simulink model "simLink_linefollower"  (R2022b)
settings: Solver=FixedStepAuto  StartTime=0.0  StopTime=10  FixedStep=0.1  RelTol=1e-3
values from neighbouring files (symbols this model uses):
  length_body = pixel_body/pixel_conversion    (= 80)    [startSim.m]
  length_close_sensor = pixel_body/pixel_conversion    (= 80)    [startSim.m]
  map = zeros(map_size_x, map_size_y)    [generate_map.m]    (also in startSim.m = imcomplement(map))
  pixel_sensor = 3    [startSim.m]
  Position_noise = 0    [startSim.m]
  reading_noise = 0    [startSim.m]
  spacing = 2/pixel_conversion    (= 20)    [startSim.m]
  velocity_left = 80    [startSim.m]
  velocity_right = 80    [startSim.m]
undefined symbols (not defined in the file or in its folder): offset_x, offset_y
libraries: simulink x28, slpidlib x1, robotmobilelib x1
(part 1 of 2)
settings Model: Creator=andre  LastModifiedBy=andre

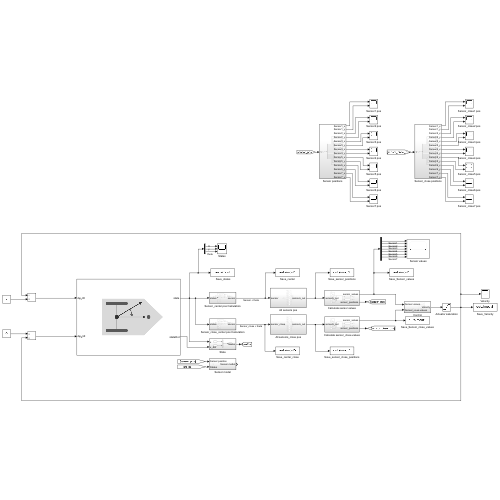
[thumbnail: Simulink's stored preview of the top-level diagram]
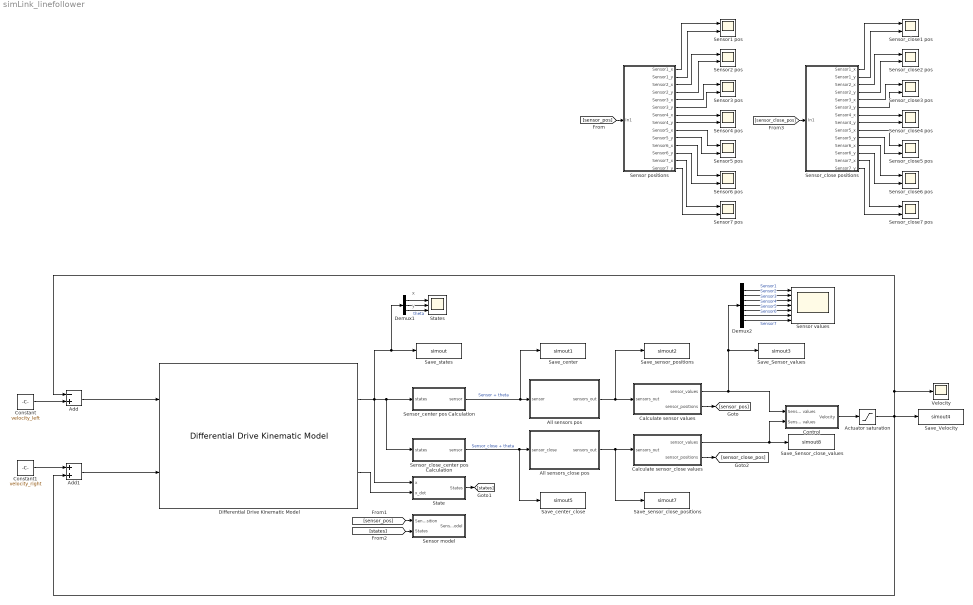
== system simLink_linefollower ==
  note: y
  note: x
  " Save_states" : ToWorkspace  VariableName=simout  SaveFormat=Structure With Time  SampleTime=-1
  Actuator saturation : Saturate  UpperLimit=velocity_left*2  LowerLimit=-velocity_left*2
  Add : Sum  Inputs=-+
  Add1 : Sum
  All sensors pos : Subsystem
  All sensors_close pos : Subsystem
  Calculate sensor values : Subsystem
  Calculate sensor_close values : Subsystem
  Constant : Constant  Value=velocity_left
  Constant1 : Constant  Value=velocity_right
  Control : Subsystem
  Demux1 : Demux  Outputs=3
  Demux2 : Demux  Outputs=7
  Differential Drive Kinematic Model : robotmobilelib/Differential Drive Kinematic Model  VehicleInputs=Wheel Speeds  WheelRadius=length_body*0.1  WheelSpeedRange=[-inf inf]  TrackWidth=length_body*0.7  InitialState=initialState  SimulateUsing=Interpreted execution
  Save_Sensor_close_values : ToWorkspace  VariableName=simout8  SaveFormat=Structure With Time  SampleTime=-1
  Save_Sensor_values : ToWorkspace  VariableName=simout3  SaveFormat=Structure With Time  SampleTime=-1
  Save_Velocity : ToWorkspace  VariableName=simout4  SaveFormat=Structure With Time  SampleTime=-1
  Save_center : ToWorkspace  VariableName=simout1  SaveFormat=Structure With Time  SampleTime=-1
  Save_center_close : ToWorkspace  VariableName=simout5  SaveFormat=Structure With Time  SampleTime=-1
  Save_sensor_close_positions : ToWorkspace  VariableName=simout7  SaveFormat=Structure With Time  SampleTime=-1
  Save_sensor_positions : ToWorkspace  VariableName=simout2  SaveFormat=Structure With Time  SampleTime=-1
  Sensor model : Subsystem
  Sensor positions : Subsystem
  Sensor values : Scope  NumInputPorts=7
  Sensor1 pos : Scope  NumInputPorts=2
  Sensor2 pos : Scope  NumInputPorts=2
  Sensor3 pos : Scope  NumInputPorts=2
  Sensor4 pos : Scope  NumInputPorts=2
  Sensor5 pos : Scope  NumInputPorts=2
  Sensor6 pos : Scope  NumInputPorts=2
  Sensor7 pos : Scope  NumInputPorts=2
  Sensor_center pos Calculation : Subsystem
  Sensor_close positions : Subsystem
  Sensor_close1 pos : Scope  NumInputPorts=2
  Sensor_close2 pos : Scope  NumInputPorts=2
  Sensor_close3 pos : Scope  NumInputPorts=2
  Sensor_close4 pos : Scope  NumInputPorts=2
  Sensor_close5 pos : Scope  NumInputPorts=2
  Sensor_close6 pos : Scope  NumInputPorts=2
  Sensor_close7 pos : Scope  NumInputPorts=2
  Sensor_close_center pos Calculation : Subsystem
  State : Subsystem
  States : Scope  NumInputPorts=3
  Velocity : Scope
  wires:
  Sensor_center pos Calculation/1(sensor) -> Save_center/1, All sensors pos/1(sensor)  "Sensor + theta"
  Differential Drive Kinematic Model/1 -> Demux1/1, " Save_states"/1, State/1(x), Sensor_close_center pos Calculation/1(states), Sensor_center pos Calculation/1(states)
  All sensors pos/1(sensors_out) -> Calculate sensor values/1(sensors_out), Save_sensor_positions/1
  Control/1(Velocity) -> Actuator saturation/1
  Constant/1 -> Add/2
  Constant1/1 -> Add1/1
  Add1/1 -> Differential Drive Kinematic Model/2
  Add/1 -> Differential Drive Kinematic Model/1
  Demux1/1 -> States/1
  Demux1/2 -> States/2
  Demux1/3 -> States/3  "theta"
  Calculate sensor values/1(sensor_values) -> Control/1(Sensor values), Demux2/1, Save_Sensor_values/1
  Demux2/1 -> Sensor values/1  "Sensor1"
  Demux2/2 -> Sensor values/2  "Sensor2"
  Demux2/3 -> Sensor values/3  "Sensor3"
  Demux2/4 -> Sensor values/4  "Sensor4"
  Demux2/5 -> Sensor values/5  "Sensor5"
  Demux2/6 -> Sensor values/6  "Sensor6"
  Demux2/7 -> Sensor values/7  "Sensor7"
  [sensor_pos] -> Sensor positions/1(In1)
  Sensor positions/1(Sensor1_x) -> Sensor1 pos/1
  Sensor positions/2(Sensor1_y) -> Sensor1 pos/2
  Sensor positions/3(Sensor2_x) -> Sensor2 pos/1
  Sensor positions/4(Sensor2_y) -> Sensor2 pos/2
  Sensor positions/5(Sensor3_x) -> Sensor3 pos/1
  Sensor positions/6(Sensor3_y) -> Sensor3 pos/2
  Sensor positions/7(Sensor4_x) -> Sensor4 pos/1
  Sensor positions/8(Sensor4_y) -> Sensor4 pos/2
  Sensor positions/9(Sensor5_x) -> Sensor5 pos/1
  Sensor positions/10(Sensor5_y) -> Sensor5 pos/2
  Sensor positions/11(Sensor6_x) -> Sensor6 pos/1
  Sensor positions/12(Sensor6_y) -> Sensor6 pos/2
  Sensor positions/13(Sensor7_x) -> Sensor7 pos/1
  Sensor positions/14(Sensor7_y) -> Sensor7 pos/2
  Calculate sensor values/2(sensor_positions) -> [sensor_pos]
  Actuator saturation/1 -> Add/1, Velocity/1, Save_Velocity/1, Add1/2
  Sensor_close_center pos Calculation/1(sensor) -> Save_center_close/1, All sensors_close pos/1(sensor_close)  "Sensor_close + theta"
  Sensor_close positions/2(Sensor1_y) -> Sensor_close1 pos/2
  Sensor_close positions/4(Sensor2_y) -> Sensor_close2 pos/2
  Sensor_close positions/7(Sensor4_x) -> Sensor_close4 pos/1
  Sensor_close positions/3(Sensor2_x) -> Sensor_close2 pos/1
  Sensor_close positions/6(Sensor3_y) -> Sensor_close3 pos/2
  Sensor_close positions/8(Sensor4_y) -> Sensor_close4 pos/2
  Sensor_close positions/13(Sensor7_x) -> Sensor_close7 pos/1
  Sensor_close positions/1(Sensor1_x) -> Sensor_close1 pos/1
  Sensor_close positions/9(Sensor5_x) -> Sensor_close5 pos/1
  Sensor_close positions/14(Sensor7_y) -> Sensor_close7 pos/2
  Sensor_close positions/11(Sensor6_x) -> Sensor_close6 pos/1
  Sensor_close positions/12(Sensor6_y) -> Sensor_close6 pos/2
  [sensor_close_pos] -> Sensor_close positions/1(In1)
  Sensor_close positions/10(Sensor5_y) -> Sensor_close5 pos/2
  Sensor_close positions/5(Sensor3_x) -> Sensor_close3 pos/1
  All sensors_close pos/1(sensors_out) -> Save_sensor_close_positions/1, Calculate sensor_close values/1(sensors_out)
  Calculate sensor_close values/2(sensor_positions) -> [sensor_close_pos]
  Calculate sensor_close values/1(sensor_values) -> Control/2(Sensor_close values), Save_Sensor_close_values/1
  Differential Drive Kinematic Model/2 -> State/2(x_dot)
  [sensor_pos] -> Sensor model/1(Sensor position)
  State/1(States) -> [states]
  [states] -> Sensor model/2(States)

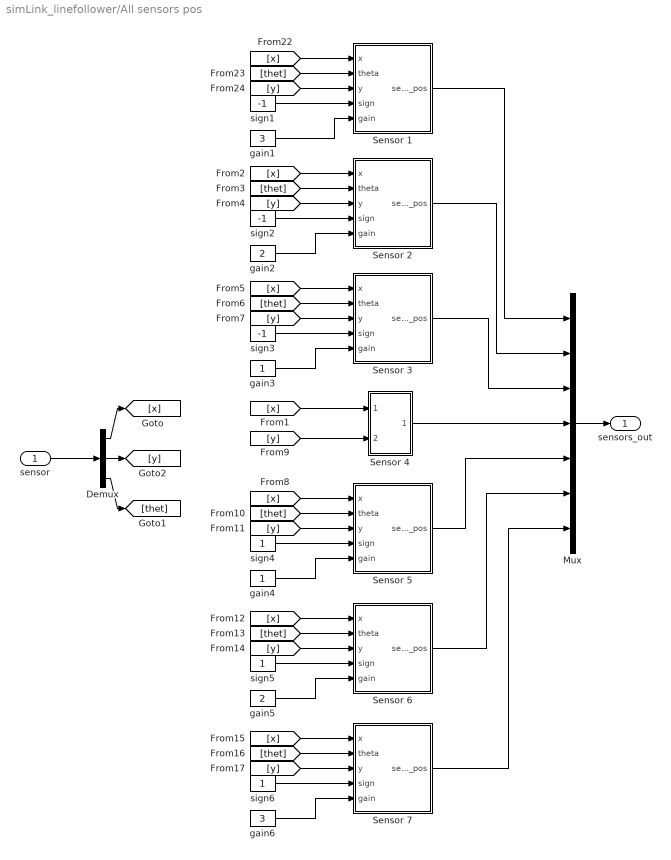
== system simLink_linefollower/All sensors pos ==
  sensor : Inport
  Demux : Demux  Outputs=3
  Mux : Mux  Inputs=7
  Sensor 1 : Subsystem
  Sensor 2 : Subsystem
  Sensor 3 : Subsystem
  Sensor 4 : Subsystem
  Sensor 5 : Subsystem
  Sensor 6 : Subsystem
  Sensor 7 : Subsystem
  gain1 : Constant  Value=3
  gain2 : Constant  Value=2
  gain3 : Constant
  gain4 : Constant
  gain5 : Constant  Value=2
  gain6 : Constant  Value=3
  sign1 : Constant  Value=-1
  sign2 : Constant  Value=-1
  sign3 : Constant  Value=-1
  sign4 : Constant
  sign5 : Constant
  sign6 : Constant
  sensors_out : Outport
  wires:
  sensor/1 -> Demux/1
  Demux/1 -> [x]
  Demux/2 -> [y]
  Mux/1 -> sensors_out/1
  [x] -> Sensor 1/1(x)
  [thet] -> Sensor 1/2(theta)
  [y] -> Sensor 1/3(y)
  Sensor 1/1(sensor_pos) -> Mux/1
  [x] -> Sensor 4/1(In1)
  [y] -> Sensor 4/2(In2)
  Sensor 4/1(Out1) -> Mux/4
  sign1/1 -> Sensor 1/4(sign)
  gain1/1 -> Sensor 1/5(gain)
  [x] -> Sensor 2/1(x)
  [x] -> Sensor 3/1(x)
  [x] -> Sensor 5/1(x)
  [thet] -> Sensor 5/2(theta)
  [x] -> Sensor 6/1(x)
  [x] -> Sensor 7/1(x)
  Sensor 2/1(sensor_pos) -> Mux/2
  Sensor 3/1(sensor_pos) -> Mux/3
  Sensor 5/1(sensor_pos) -> Mux/5
  Sensor 6/1(sensor_pos) -> Mux/6
  Sensor 7/1(sensor_pos) -> Mux/7
  [thet] -> Sensor 2/2(theta)
  [y] -> Sensor 2/3(y)
  sign2/1 -> Sensor 2/4(sign)
  gain2/1 -> Sensor 2/5(gain)
  [thet] -> Sensor 3/2(theta)
  [y] -> Sensor 3/3(y)
  gain3/1 -> Sensor 3/5(gain)
  sign3/1 -> Sensor 3/4(sign)
  [y] -> Sensor 5/3(y)
  sign4/1 -> Sensor 5/4(sign)
  gain4/1 -> Sensor 5/5(gain)
  [thet] -> Sensor 6/2(theta)
  [y] -> Sensor 6/3(y)
  sign5/1 -> Sensor 6/4(sign)
  gain5/1 -> Sensor 6/5(gain)
  [thet] -> Sensor 7/2(theta)
  [y] -> Sensor 7/3(y)
  sign6/1 -> Sensor 7/4(sign)
  gain6/1 -> Sensor 7/5(gain)
  Demux/3 -> [thet]

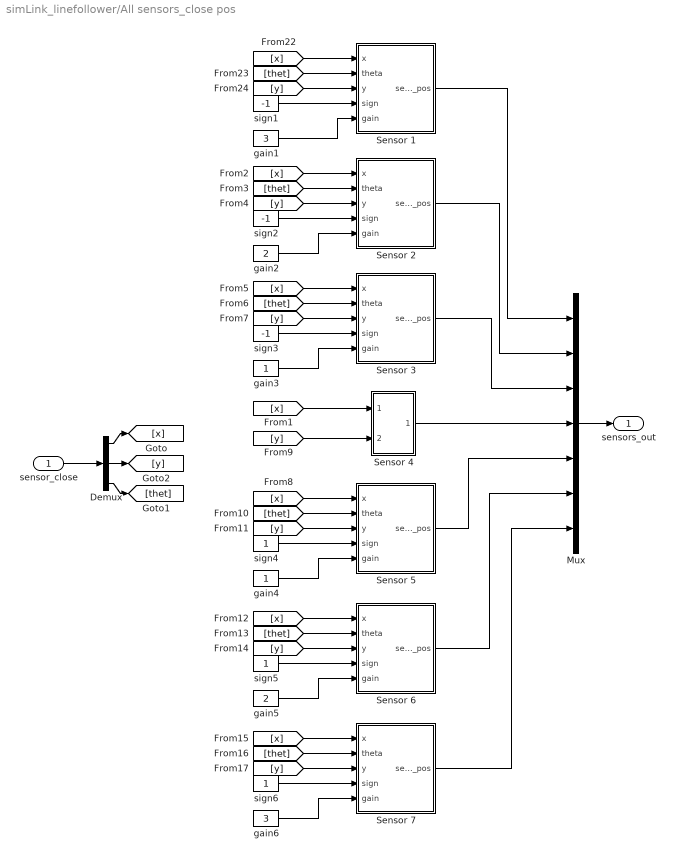
== system simLink_linefollower/All sensors_close pos ==
  sensor_close : Inport
  Demux : Demux  Outputs=3
  Mux : Mux  Inputs=7
  Sensor 1 : Subsystem
  Sensor 2 : Subsystem
  Sensor 3 : Subsystem
  Sensor 4 : Subsystem
  Sensor 5 : Subsystem
  Sensor 6 : Subsystem
  Sensor 7 : Subsystem
  gain1 : Constant  Value=3
  gain2 : Constant  Value=2
  gain3 : Constant
  gain4 : Constant
  gain5 : Constant  Value=2
  gain6 : Constant  Value=3
  sign1 : Constant  Value=-1
  sign2 : Constant  Value=-1
  sign3 : Constant  Value=-1
  sign4 : Constant
  sign5 : Constant
  sign6 : Constant
  sensors_out : Outport
  wires:
  sensor_close/1 -> Demux/1
  Demux/1 -> [x]
  Demux/2 -> [y]
  Mux/1 -> sensors_out/1
  [x] -> Sensor 1/1(x)
  [thet] -> Sensor 1/2(theta)
  [y] -> Sensor 1/3(y)
  Sensor 1/1(sensor_pos) -> Mux/1
  [x] -> Sensor 4/1(In1)
  [y] -> Sensor 4/2(In2)
  Sensor 4/1(Out1) -> Mux/4
  sign1/1 -> Sensor 1/4(sign)
  gain1/1 -> Sensor 1/5(gain)
  [x] -> Sensor 2/1(x)
  [x] -> Sensor 3/1(x)
  [x] -> Sensor 5/1(x)
  [thet] -> Sensor 5/2(theta)
  [x] -> Sensor 6/1(x)
  [x] -> Sensor 7/1(x)
  Sensor 2/1(sensor_pos) -> Mux/2
  Sensor 3/1(sensor_pos) -> Mux/3
  Sensor 5/1(sensor_pos) -> Mux/5
  Sensor 6/1(sensor_pos) -> Mux/6
  Sensor 7/1(sensor_pos) -> Mux/7
  [thet] -> Sensor 2/2(theta)
  [y] -> Sensor 2/3(y)
  sign2/1 -> Sensor 2/4(sign)
  gain2/1 -> Sensor 2/5(gain)
  [thet] -> Sensor 3/2(theta)
  [y] -> Sensor 3/3(y)
  gain3/1 -> Sensor 3/5(gain)
  sign3/1 -> Sensor 3/4(sign)
  [y] -> Sensor 5/3(y)
  sign4/1 -> Sensor 5/4(sign)
  gain4/1 -> Sensor 5/5(gain)
  [thet] -> Sensor 6/2(theta)
  [y] -> Sensor 6/3(y)
  sign5/1 -> Sensor 6/4(sign)
  gain5/1 -> Sensor 6/5(gain)
  [thet] -> Sensor 7/2(theta)
  [y] -> Sensor 7/3(y)
  sign6/1 -> Sensor 7/4(sign)
  gain6/1 -> Sensor 7/5(gain)
  Demux/3 -> [thet]

== system simLink_linefollower/Calculate sensor values ==
  sensors_out : Inport
  Add noise to values : Subsystem
  Added noise to positions : Subsystem
  Image : Constant  Value=map
  MATLAB Function : MATLAB Function  TreatAsAtomicUnit=on
  Number of sensor pixels : Constant  Value=pixel_sensor
  Offset for x : Constant  Value=offset_x
  Offset for y : Constant  Value=offset_y
  sensor_values : Outport
  sensor_positions : Outport  Port=2
  wires:
  sensors_out/1 -> MATLAB Function/1(coord)
  MATLAB Function/1(sensor_values) -> Add noise to values/1(Values)
  Image/1 -> MATLAB Function/2(img)
  Offset for x/1 -> MATLAB Function/3(offset_x)
  Offset for y/1 -> MATLAB Function/4(offset_y)
  Number of sensor pixels/1 -> MATLAB Function/5(pixel)
  MATLAB Function/2(pos) -> Added noise to positions/1(Position)
  Add noise to values/1(Out1) -> sensor_values/1
  Added noise to positions/1(sensor_positions) -> sensor_positions/1

== system simLink_linefollower/Calculate sensor_close values ==
  sensors_out : Inport
  Add noise to values : Subsystem
  Added noise to positions : Subsystem
  Image : Constant  Value=map
  MATLAB Function : MATLAB Function  TreatAsAtomicUnit=on
  Number of sensor pixels : Constant  Value=pixel_sensor
  Offset for x : Constant  Value=offset_x
  Offset for y : Constant  Value=offset_y
  sensor_values : Outport
  sensor_positions : Outport  Port=2
  wires:
  sensors_out/1 -> MATLAB Function/1(coord)
  MATLAB Function/1(sensor_values) -> Add noise to values/1(Values)
  Image/1 -> MATLAB Function/2(img)
  Offset for x/1 -> MATLAB Function/3(offset_x)
  Offset for y/1 -> MATLAB Function/4(offset_y)
  Number of sensor pixels/1 -> MATLAB Function/5(pixel)
  MATLAB Function/2(pos) -> Added noise to positions/1(Position)
  Add noise to values/1(Out1) -> sensor_values/1
  Added noise to positions/1(sensor_positions) -> sensor_positions/1

== system simLink_linefollower/Control ==
  note: Sensor sum
  note: Error
  Sensor values : Inport
  Sensor_close values : Inport  Port=2
  Add and scale sensor values : Subsystem
  BaseLine : Constant  Value=0
  Baseline : Constant  Value=0
  Error : Scope  NumInputPorts=2
  PID Controller : slpidlib/PID Controller  Controller=PID  Form=Parallel  TimeDomain=Continuous-time  UseExternalTs=off  SampleTime=-1  IntegratorMethod=Forward Euler  FilterMethod=Forward Euler  ControllerParametersSource=internal  P=0.2  I=1  UseKiTs=off  D=0  N=100  UseFilter=on  TunerSelectOption=Transfer Function Based (PID Tuner App)  InitialConditionSource=internal  InitialConditionForIntegrator=0  InitialConditionForFilter=0  DifferentiatorICPrevScaledInput=0  ExternalReset=none  TrackingMode=off  Kt=1  LimitOutput=off  SatLimitsSource=internal  UpperSaturationLimit=inf  LowerSaturationLimit=-inf  LinearizeAsGain=on  AntiWindupMode=none  Kb=1  LimitIntegrator=off  UpperIntegratorSaturationLimit=inf  LowerIntegratorSaturationLimit=-inf  POutMin=[]  POutMax=[]  IOutMin=[]  IOutMax=[]  DOutMin=[]  DOutMax=[]  NOutMin=[]  NOutMax=[]  SumOutMin=[]  SumOutMax=[]  SaturationOutMin=[]  SaturationOutMax=[]  PParamMin=[]  PParamMax=[]  IParamMin=[]  IParamMax=[]  DParamMin=[]  DParamMax=[]  NParamMin=[]  NParamMax=[]  KbParamMin=[]  KbParamMax=[]  KtParamMin=[]  KtParamMax=[]  KbOutMin=[]  KbOutMax=[]  KtOutMin=[]  KtOutMax=[]  IntegratorOutMin=[]  IntegratorOutMax=[]  FilterOutMin=[]  FilterOutMax=[]  SumI1OutMin=[]  SumI1OutMax=[]  SumI2OutMin=[]  SumI2OutMax=[]  SumI3OutMin=[]  SumI3OutMax=[]  SumI4OutMin=[]  SumI4OutMax=[]  SumDOutMin=[]  SumDOutMax=[]  DifferentiatorOutMin=[]  DifferentiatorOutMax=[]  FilterDiffOutCoefMin=[]  FilterDiffOutCoefMax=[]  ReciprocalOutMin=[]  ReciprocalOutMax=[]  SumDenOutMin=[]  SumDenOutMax=[]  SumNumOutMin=[]  SumNumOutMax=[]  DivideOutMin=[]  DivideOutMax=[]  UdiffTsProdOutMin=[]  UdiffTsProdOutMax=[]  NTsProdOutMin=[]  NTsProdOutMax=[]  UintegralTsProdOutMin=[]  UintegralTsProdOutMax=[]  UngainTsProdOutMin=[]  UngainTsProdOutMax=[]  ClampingZeroOutDataTypeStr=Inherit: Inherit via back propagation  ClampingZeroOutMin=[]  ClampingZeroOutMax=[]  FilterDenConstantOutDataTypeStr=Inherit: Inherit via back propagation  FilterDenConstantOutMin=[]  FilterDenConstantOutMax=[]  PCopyOutDataTypeStr=Inherit: Inherit via back propagation  PCopyOutMin=[]  PCopyOutMax=[]  NCopyOutDataTypeStr=Inherit: Inherit via back propagation  NCopyOutMin=[]  NCopyOutMax=[]  IntegratorContinuousStateAttributes=''  IntegratorStateMustResolveToSignalObject=off  IntegratorRTWStateStorageClass=Auto  FilterContinuousStateAttributes=''  FilterStateMustResolveToSignalObject=off  FilterRTWStateStorageClass=Auto  ParallelPVariant=InternalParameters  IdealPVariant=Disabled  IVariant=InternalParameters  DVariant=InternalParameters  IntegratorVariant=Continuous  SatVariant=Disabled  AWVariant=Passthrough  PCopyVariant=Disabled  TRVariant=Disabled  FdbkBlocksVariant=Forward  IdealPFdbkVariant=Disabled  SatFdbkVariant=Disabled  DerivativeFilterVariant=ContFilter  NVariant=InternalParameters  NCopyVariant=Disabled  FilterICVariant=InternalICsFilter  IntegratorICVariant=InternalICs  ExternalResetVariant=Disabled  TRSumVariant=Passthrough  SumFdbkVariant=Disabled  SumVariant=Sum_PID  TsampFilterVariant=InternalTs  TsampNgainVariant=Passthrough  TsampIntegralVariant=Passthrough  ExternalSaturationOutDataTypeStr=Inherit: Same as second input
  Sensor_close_values : Scope
  Sensor_sum : Scope
  Sensor_values : Scope
  Subtract : Sum  Inputs=+-
  Velocity : Outport
  wires:
  Sensor values/1 -> [Sensor_values], Add and scale sensor values/1(Sensor values)
  Baseline/1 -> Subtract/1
  Subtract/1 -> Error/1, PID Controller/1
  PID Controller/1 -> Velocity/1
  BaseLine/1 -> Error/2
  [Sensor_close_values] -> Sensor_close_values/1
  [Sensor_values] -> Sensor_values/1
  Sensor_close values/1 -> [Sensor_close_values], Add and scale sensor values/2(Sensor_close values)
  Add and scale sensor values/1(Sensor sum) -> Subtract/2, Sensor_sum/1

== system simLink_linefollower/Sensor model ==
  Sensor position : Inport
  States : Inport  Port=2
  Sensor model : Outport

== system simLink_linefollower/Sensor positions ==
  In1 : Inport
  Demux3 : Demux  Outputs=14
  Sensor1_x : Outport
  Sensor1_y : Outport  Port=2
  Sensor2_x : Outport  Port=3
  Sensor2_y : Outport  Port=4
  Sensor3_x : Outport  Port=5
  Sensor3_y : Outport  Port=6
  Sensor4_x : Outport  Port=7
  Sensor4_y : Outport  Port=8
  Sensor5_x : Outport  Port=9
  Sensor5_y : Outport  Port=10
  Sensor6_x : Outport  Port=11
  Sensor6_y : Outport  Port=12
  Sensor7_x : Outport  Port=13
  Sensor7_y : Outport  Port=14
  wires:
  Demux3/5 -> Sensor3_x/1  "Sensor3_x"
  Demux3/3 -> Sensor2_x/1  "Sensor2_x"
  Demux3/7 -> Sensor4_x/1  "Sensor4_x"
  Demux3/8 -> Sensor4_y/1  "Sensor4_y"
  Demux3/12 -> Sensor6_y/1  "Sensor6_y"
  Demux3/4 -> Sensor2_y/1  "Sensor2_y"
  Demux3/1 -> Sensor1_x/1  "Sensor1_x"
  Demux3/13 -> Sensor7_x/1  "Sensor7_x"
  In1/1 -> Demux3/1
  Demux3/6 -> Sensor3_y/1  "Sensor3_y"
  Demux3/14 -> Sensor7_y/1  "Sensor7_y"
  Demux3/2 -> Sensor1_y/1  "Sensor1_y"
  Demux3/11 -> Sensor6_x/1  "Sensor6_x"
  Demux3/10 -> Sensor5_y/1  "Sensor5_y"
  Demux3/9 -> Sensor5_x/1  "Sensor5_x"

== system simLink_linefollower/Sensor_center pos Calculation ==
  states : Inport
  Add : Sum
  Add1 : Sum
  Demux : Demux  Outputs=3
  Length body1 : Gain  Gain=length_body
  Length body2 : Gain  Gain=length_body
  Mux : Mux  Inputs=3
  Sin : Trigonometry
  Sin1 : Trigonometry  Operator=cos
  theta : Scope
  sensor : Outport
  wires:
  Mux/1 -> sensor/1
  Length body1/1 -> Add/2
  Demux/1 -> Add1/1
  Sin/1 -> Length body1/1
  Demux/3 -> [theta], theta/1, Sin1/1, Sin/1
  Length body2/1 -> Add1/2
  Sin1/1 -> Length body2/1
  Demux/2 -> Add/1
  states/1 -> Demux/1
  Add1/1 -> Mux/1
  Add/1 -> Mux/2
  [theta] -> Mux/3

== system simLink_linefollower/Sensor_close positions ==
  In1 : Inport
  Demux3 : Demux  Outputs=14
  Sensor1_x : Outport
  Sensor1_y : Outport  Port=2
  Sensor2_x : Outport  Port=3
  Sensor2_y : Outport  Port=4
  Sensor3_x : Outport  Port=5
  Sensor3_y : Outport  Port=6
  Sensor4_x : Outport  Port=7
  Sensor4_y : Outport  Port=8
  Sensor5_x : Outport  Port=9
  Sensor5_y : Outport  Port=10
  Sensor6_x : Outport  Port=11
  Sensor6_y : Outport  Port=12
  Sensor7_x : Outport  Port=13
  Sensor7_y : Outport  Port=14
  wires:
  Demux3/5 -> Sensor3_x/1  "Sensor3_x"
  Demux3/3 -> Sensor2_x/1  "Sensor2_x"
  Demux3/7 -> Sensor4_x/1  "Sensor4_x"
  Demux3/8 -> Sensor4_y/1  "Sensor4_y"
  Demux3/12 -> Sensor6_y/1  "Sensor6_y"
  Demux3/4 -> Sensor2_y/1  "Sensor2_y"
  Demux3/1 -> Sensor1_x/1  "Sensor1_x"
  Demux3/13 -> Sensor7_x/1  "Sensor7_x"
  In1/1 -> Demux3/1
  Demux3/6 -> Sensor3_y/1  "Sensor3_y"
  Demux3/14 -> Sensor7_y/1  "Sensor7_y"
  Demux3/2 -> Sensor1_y/1  "Sensor1_y"
  Demux3/11 -> Sensor6_x/1  "Sensor6_x"
  Demux3/10 -> Sensor5_y/1  "Sensor5_y"
  Demux3/9 -> Sensor5_x/1  "Sensor5_x"

== system simLink_linefollower/Sensor_close_center pos Calculation ==
  states : Inport
  Add : Sum
  Add1 : Sum
  Demux : Demux  Outputs=3
  Length body1 : Gain  Gain=length_close_sensor
  Length body2 : Gain  Gain=length_close_sensor
  Mux : Mux  Inputs=3
  Sin : Trigonometry
  Sin1 : Trigonometry  Operator=cos
  theta : Scope
  sensor : Outport
  wires:
  Mux/1 -> sensor/1
  Length body1/1 -> Add/2
  Demux/1 -> Add1/1
  Sin/1 -> Length body1/1
  Demux/3 -> [theta], theta/1, Sin1/1, Sin/1
  Length body2/1 -> Add1/2
  Sin1/1 -> Length body2/1
  Demux/2 -> Add/1
  states/1 -> Demux/1
  Add1/1 -> Mux/1
  Add/1 -> Mux/2
  [theta] -> Mux/3

== system simLink_linefollower/State ==
  x : Inport
  x_dot : Inport  Port=2
  Mux : Mux  Inputs=2
  States : Outport
  wires:
  x/1 -> Mux/1
  x_dot/1 -> Mux/2
  Mux/1 -> States/1

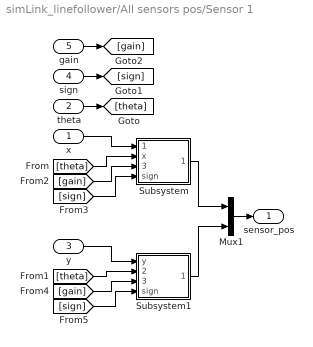
== system simLink_linefollower/All sensors pos/Sensor 1 ==
  x : Inport
  theta : Inport  Port=2
  y : Inport  Port=3
  sign : Inport  Port=4
  gain : Inport  Port=5
  Mux1 : Mux  Inputs=2
  Subsystem : Subsystem
  Subsystem1 : Subsystem
  sensor_pos : Outport
  wires:
  x/1 -> Subsystem/1(theta)
  Mux1/1 -> sensor_pos/1
  Subsystem1/1(y_pos) -> Mux1/2
  Subsystem/1(x_pos) -> Mux1/1
  theta/1 -> [theta]
  y/1 -> Subsystem1/1(y)
  [theta] -> Subsystem/2(x)
  [theta] -> Subsystem1/2(theta)
  sign/1 -> [sign]
  gain/1 -> [gain]
  [gain] -> Subsystem/3(gain)
  [sign] -> Subsystem/4(sign)
  [gain] -> Subsystem1/3(gain)
  [sign] -> Subsystem1/4(sign)

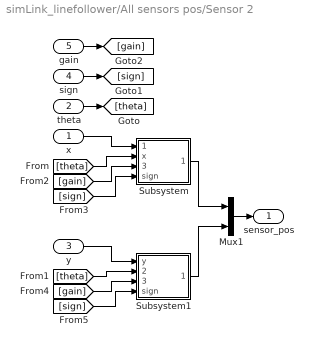
== system simLink_linefollower/All sensors pos/Sensor 2 ==
  x : Inport
  theta : Inport  Port=2
  y : Inport  Port=3
  sign : Inport  Port=4
  gain : Inport  Port=5
  Mux1 : Mux  Inputs=2
  Subsystem : Subsystem
  Subsystem1 : Subsystem
  sensor_pos : Outport
  wires:
  x/1 -> Subsystem/1(theta)
  Mux1/1 -> sensor_pos/1
  Subsystem1/1(y_pos) -> Mux1/2
  Subsystem/1(x_pos) -> Mux1/1
  theta/1 -> [theta]
  y/1 -> Subsystem1/1(y)
  [theta] -> Subsystem/2(x)
  [theta] -> Subsystem1/2(theta)
  sign/1 -> [sign]
  gain/1 -> [gain]
  [gain] -> Subsystem/3(gain)
  [sign] -> Subsystem/4(sign)
  [gain] -> Subsystem1/3(gain)
  [sign] -> Subsystem1/4(sign)

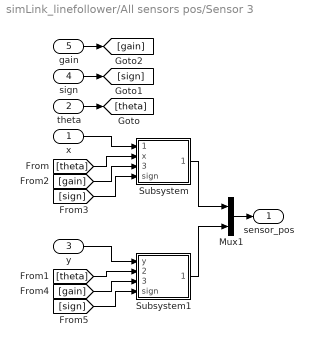
== system simLink_linefollower/All sensors pos/Sensor 3 ==
  x : Inport
  theta : Inport  Port=2
  y : Inport  Port=3
  sign : Inport  Port=4
  gain : Inport  Port=5
  Mux1 : Mux  Inputs=2
  Subsystem : Subsystem
  Subsystem1 : Subsystem
  sensor_pos : Outport
  wires:
  x/1 -> Subsystem/1(theta)
  Mux1/1 -> sensor_pos/1
  Subsystem1/1(y_pos) -> Mux1/2
  Subsystem/1(x_pos) -> Mux1/1
  theta/1 -> [theta]
  y/1 -> Subsystem1/1(y)
  [theta] -> Subsystem/2(x)
  [theta] -> Subsystem1/2(theta)
  sign/1 -> [sign]
  gain/1 -> [gain]
  [gain] -> Subsystem/3(gain)
  [sign] -> Subsystem/4(sign)
  [gain] -> Subsystem1/3(gain)
  [sign] -> Subsystem1/4(sign)

== system simLink_linefollower/All sensors pos/Sensor 4 ==
  In1 : Inport
  In2 : Inport  Port=2
  Mux4 : Mux  Inputs=2
  Out1 : Outport
  wires:
  In2/1 -> Mux4/2
  In1/1 -> Mux4/1
  Mux4/1 -> Out1/1

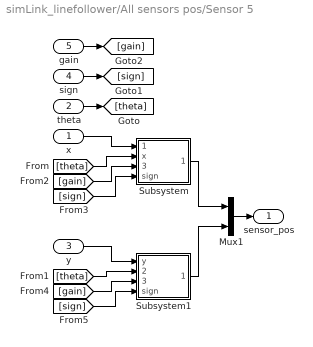
== system simLink_linefollower/All sensors pos/Sensor 5 ==
  x : Inport
  theta : Inport  Port=2
  y : Inport  Port=3
  sign : Inport  Port=4
  gain : Inport  Port=5
  Mux1 : Mux  Inputs=2
  Subsystem : Subsystem
  Subsystem1 : Subsystem
  sensor_pos : Outport
  wires:
  x/1 -> Subsystem/1(theta)
  Mux1/1 -> sensor_pos/1
  Subsystem1/1(y_pos) -> Mux1/2
  Subsystem/1(x_pos) -> Mux1/1
  theta/1 -> [theta]
  y/1 -> Subsystem1/1(y)
  [theta] -> Subsystem/2(x)
  [theta] -> Subsystem1/2(theta)
  sign/1 -> [sign]
  gain/1 -> [gain]
  [gain] -> Subsystem/3(gain)
  [sign] -> Subsystem/4(sign)
  [gain] -> Subsystem1/3(gain)
  [sign] -> Subsystem1/4(sign)

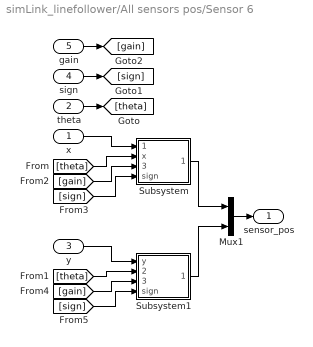
== system simLink_linefollower/All sensors pos/Sensor 6 ==
  x : Inport
  theta : Inport  Port=2
  y : Inport  Port=3
  sign : Inport  Port=4
  gain : Inport  Port=5
  Mux1 : Mux  Inputs=2
  Subsystem : Subsystem
  Subsystem1 : Subsystem
  sensor_pos : Outport
  wires:
  x/1 -> Subsystem/1(theta)
  Mux1/1 -> sensor_pos/1
  Subsystem1/1(y_pos) -> Mux1/2
  Subsystem/1(x_pos) -> Mux1/1
  theta/1 -> [theta]
  y/1 -> Subsystem1/1(y)
  [theta] -> Subsystem/2(x)
  [theta] -> Subsystem1/2(theta)
  sign/1 -> [sign]
  gain/1 -> [gain]
  [gain] -> Subsystem/3(gain)
  [sign] -> Subsystem/4(sign)
  [gain] -> Subsystem1/3(gain)
  [sign] -> Subsystem1/4(sign)

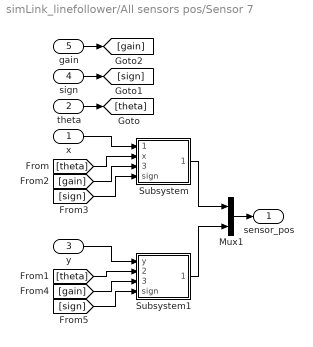
== system simLink_linefollower/All sensors pos/Sensor 7 ==
  x : Inport
  theta : Inport  Port=2
  y : Inport  Port=3
  sign : Inport  Port=4
  gain : Inport  Port=5
  Mux1 : Mux  Inputs=2
  Subsystem : Subsystem
  Subsystem1 : Subsystem
  sensor_pos : Outport
  wires:
  x/1 -> Subsystem/1(theta)
  Mux1/1 -> sensor_pos/1
  Subsystem1/1(y_pos) -> Mux1/2
  Subsystem/1(x_pos) -> Mux1/1
  theta/1 -> [theta]
  y/1 -> Subsystem1/1(y)
  [theta] -> Subsystem/2(x)
  [theta] -> Subsystem1/2(theta)
  sign/1 -> [sign]
  gain/1 -> [gain]
  [gain] -> Subsystem/3(gain)
  [sign] -> Subsystem/4(sign)
  [gain] -> Subsystem1/3(gain)
  [sign] -> Subsystem1/4(sign)

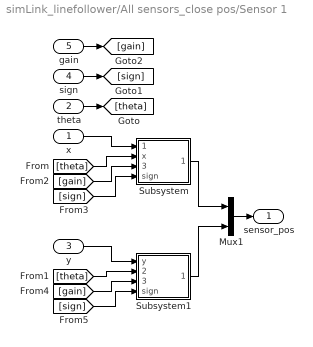
== system simLink_linefollower/All sensors_close pos/Sensor 1 ==
  x : Inport
  theta : Inport  Port=2
  y : Inport  Port=3
  sign : Inport  Port=4
  gain : Inport  Port=5
  Mux1 : Mux  Inputs=2
  Subsystem : Subsystem
  Subsystem1 : Subsystem
  sensor_pos : Outport
  wires:
  x/1 -> Subsystem/1(theta)
  Mux1/1 -> sensor_pos/1
  Subsystem1/1(y_pos) -> Mux1/2
  Subsystem/1(x_pos) -> Mux1/1
  theta/1 -> [theta]
  y/1 -> Subsystem1/1(y)
  [theta] -> Subsystem/2(x)
  [theta] -> Subsystem1/2(theta)
  sign/1 -> [sign]
  gain/1 -> [gain]
  [gain] -> Subsystem/3(gain)
  [sign] -> Subsystem/4(sign)
  [gain] -> Subsystem1/3(gain)
  [sign] -> Subsystem1/4(sign)

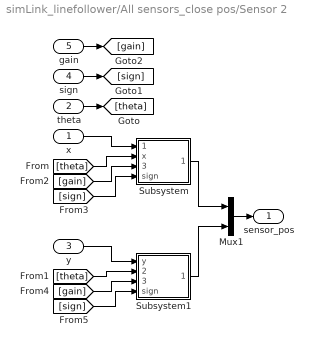
== system simLink_linefollower/All sensors_close pos/Sensor 2 ==
  x : Inport
  theta : Inport  Port=2
  y : Inport  Port=3
  sign : Inport  Port=4
  gain : Inport  Port=5
  Mux1 : Mux  Inputs=2
  Subsystem : Subsystem
  Subsystem1 : Subsystem
  sensor_pos : Outport
  wires:
  x/1 -> Subsystem/1(theta)
  Mux1/1 -> sensor_pos/1
  Subsystem1/1(y_pos) -> Mux1/2
  Subsystem/1(x_pos) -> Mux1/1
  theta/1 -> [theta]
  y/1 -> Subsystem1/1(y)
  [theta] -> Subsystem/2(x)
  [theta] -> Subsystem1/2(theta)
  sign/1 -> [sign]
  gain/1 -> [gain]
  [gain] -> Subsystem/3(gain)
  [sign] -> Subsystem/4(sign)
  [gain] -> Subsystem1/3(gain)
  [sign] -> Subsystem1/4(sign)

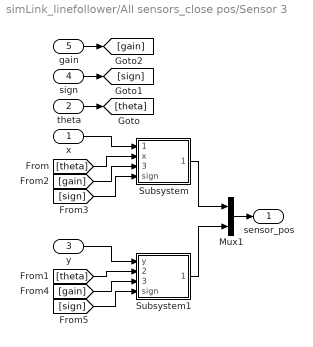
== system simLink_linefollower/All sensors_close pos/Sensor 3 ==
  x : Inport
  theta : Inport  Port=2
  y : Inport  Port=3
  sign : Inport  Port=4
  gain : Inport  Port=5
  Mux1 : Mux  Inputs=2
  Subsystem : Subsystem
  Subsystem1 : Subsystem
  sensor_pos : Outport
  wires:
  x/1 -> Subsystem/1(theta)
  Mux1/1 -> sensor_pos/1
  Subsystem1/1(y_pos) -> Mux1/2
  Subsystem/1(x_pos) -> Mux1/1
  theta/1 -> [theta]
  y/1 -> Subsystem1/1(y)
  [theta] -> Subsystem/2(x)
  [theta] -> Subsystem1/2(theta)
  sign/1 -> [sign]
  gain/1 -> [gain]
  [gain] -> Subsystem/3(gain)
  [sign] -> Subsystem/4(sign)
  [gain] -> Subsystem1/3(gain)
  [sign] -> Subsystem1/4(sign)

== system simLink_linefollower/All sensors_close pos/Sensor 4 ==
  In1 : Inport
  In2 : Inport  Port=2
  Mux4 : Mux  Inputs=2
  Out1 : Outport
  wires:
  In2/1 -> Mux4/2
  In1/1 -> Mux4/1
  Mux4/1 -> Out1/1

== system simLink_linefollower/All sensors_close pos/Sensor 5 ==
  x : Inport
  theta : Inport  Port=2
  y : Inport  Port=3
  sign : Inport  Port=4
  gain : Inport  Port=5
  Mux1 : Mux  Inputs=2
  Subsystem : Subsystem
  Subsystem1 : Subsystem
  sensor_pos : Outport
  wires:
  x/1 -> Subsystem/1(theta)
  Mux1/1 -> sensor_pos/1
  Subsystem1/1(y_pos) -> Mux1/2
  Subsystem/1(x_pos) -> Mux1/1
  theta/1 -> [theta]
  y/1 -> Subsystem1/1(y)
  [theta] -> Subsystem/2(x)
  [theta] -> Subsystem1/2(theta)
  sign/1 -> [sign]
  gain/1 -> [gain]
  [gain] -> Subsystem/3(gain)
  [sign] -> Subsystem/4(sign)
  [gain] -> Subsystem1/3(gain)
  [sign] -> Subsystem1/4(sign)

== system simLink_linefollower/All sensors_close pos/Sensor 6 ==
  x : Inport
  theta : Inport  Port=2
  y : Inport  Port=3
  sign : Inport  Port=4
  gain : Inport  Port=5
  Mux1 : Mux  Inputs=2
  Subsystem : Subsystem
  Subsystem1 : Subsystem
  sensor_pos : Outport
  wires:
  x/1 -> Subsystem/1(theta)
  Mux1/1 -> sensor_pos/1
  Subsystem1/1(y_pos) -> Mux1/2
  Subsystem/1(x_pos) -> Mux1/1
  theta/1 -> [theta]
  y/1 -> Subsystem1/1(y)
  [theta] -> Subsystem/2(x)
  [theta] -> Subsystem1/2(theta)
  sign/1 -> [sign]
  gain/1 -> [gain]
  [gain] -> Subsystem/3(gain)
  [sign] -> Subsystem/4(sign)
  [gain] -> Subsystem1/3(gain)
  [sign] -> Subsystem1/4(sign)

== system simLink_linefollower/All sensors_close pos/Sensor 7 ==
  x : Inport
  theta : Inport  Port=2
  y : Inport  Port=3
  sign : Inport  Port=4
  gain : Inport  Port=5
  Mux1 : Mux  Inputs=2
  Subsystem : Subsystem
  Subsystem1 : Subsystem
  sensor_pos : Outport
  wires:
  x/1 -> Subsystem/1(theta)
  Mux1/1 -> sensor_pos/1
  Subsystem1/1(y_pos) -> Mux1/2
  Subsystem/1(x_pos) -> Mux1/1
  theta/1 -> [theta]
  y/1 -> Subsystem1/1(y)
  [theta] -> Subsystem/2(x)
  [theta] -> Subsystem1/2(theta)
  sign/1 -> [sign]
  gain/1 -> [gain]
  [gain] -> Subsystem/3(gain)
  [sign] -> Subsystem/4(sign)
  [gain] -> Subsystem1/3(gain)
  [sign] -> Subsystem1/4(sign)

== system simLink_linefollower/Calculate sensor values/Add noise to values ==
  Values : Inport
  Add{,1..6} (7 alike) : Sum
  Band-Limited White Noise{,1..6} (7 alike) : simulink/Sources/Band-Limited White Noise  Cov=[reading_noise]  Ts=0.1  seed=[23341]
  Demux : Demux  Outputs=7
  Mux : Mux  Inputs=7
  Out1 : Outport
  wires:
  Values/1 -> Demux/1
  Demux/1 -> Add/2
  Band-Limited White Noise/1 -> Add/1
  Band-Limited White Noise1/1 -> Add1/1
  Demux/2 -> Add1/2
  Band-Limited White Noise2/1 -> Add2/1
  Demux/3 -> Add2/2
  Band-Limited White Noise3/1 -> Add3/1
  Demux/4 -> Add3/2
  Band-Limited White Noise4/1 -> Add4/1
  Demux/5 -> Add4/2
  Band-Limited White Noise5/1 -> Add5/1
  Demux/6 -> Add5/2
  Band-Limited White Noise6/1 -> Add6/1
  Demux/7 -> Add6/2
  Add/1 -> Mux/1
  Add1/1 -> Mux/2
  Add2/1 -> Mux/3
  Add3/1 -> Mux/4
  Add4/1 -> Mux/5
  Add5/1 -> Mux/6
  Add6/1 -> Mux/7
  Mux/1 -> Out1/1

== system simLink_linefollower/Calculate sensor values/Added noise to positions ==
  Position : Inport
  Add{,1..6} (7 alike) : Sum
  Band-Limited White Noise{,1..6} (7 alike) : simulink/Sources/Band-Limited White Noise  Cov=[Position_noise]  Ts=0.1  seed=[23341]
  Demux : Demux  Outputs=7
  Mux : Mux  Inputs=7
  sensor_positions : Outport
  wires:
  Band-Limited White Noise2/1 -> Add2/1
  Band-Limited White Noise6/1 -> Add6/1
  Band-Limited White Noise1/1 -> Add1/1
  Band-Limited White Noise5/1 -> Add5/1
  Add5/1 -> Mux/6
  Demux/3 -> Add2/2
  Add3/1 -> Mux/4
  Add2/1 -> Mux/3
  Add1/1 -> Mux/2
  Mux/1 -> sensor_positions/1
  Add6/1 -> Mux/7
  Band-Limited White Noise/1 -> Add/1
  Demux/1 -> Add/2
  Demux/7 -> Add6/2
  Band-Limited White Noise3/1 -> Add3/1
  Demux/6 -> Add5/2
  Add/1 -> Mux/1
  Position/1 -> Demux/1
  Demux/2 -> Add1/2
  Demux/4 -> Add3/2
  Band-Limited White Noise4/1 -> Add4/1
  Demux/5 -> Add4/2
  Add4/1 -> Mux/5

== system simLink_linefollower/Calculate sensor_close values/Add noise to values ==
  Values : Inport
  Add{,1..6} (7 alike) : Sum
  Band-Limited White Noise{,1..6} (7 alike) : simulink/Sources/Band-Limited White Noise  Cov=[reading_noise]  Ts=0.1  seed=[23341]
  Demux : Demux  Outputs=7
  Mux : Mux  Inputs=7
  Out1 : Outport
  wires:
  Values/1 -> Demux/1
  Demux/1 -> Add/2
  Band-Limited White Noise/1 -> Add/1
  Band-Limited White Noise1/1 -> Add1/1
  Demux/2 -> Add1/2
  Band-Limited White Noise2/1 -> Add2/1
  Demux/3 -> Add2/2
  Band-Limited White Noise3/1 -> Add3/1
  Demux/4 -> Add3/2
  Band-Limited White Noise4/1 -> Add4/1
  Demux/5 -> Add4/2
  Band-Limited White Noise5/1 -> Add5/1
  Demux/6 -> Add5/2
  Band-Limited White Noise6/1 -> Add6/1
  Demux/7 -> Add6/2
  Add/1 -> Mux/1
  Add1/1 -> Mux/2
  Add2/1 -> Mux/3
  Add3/1 -> Mux/4
  Add4/1 -> Mux/5
  Add5/1 -> Mux/6
  Add6/1 -> Mux/7
  Mux/1 -> Out1/1

== system simLink_linefollower/Calculate sensor_close values/Added noise to positions ==
  Position : Inport
  Add{,1..6} (7 alike) : Sum
  Band-Limited White Noise{,1..6} (7 alike) : simulink/Sources/Band-Limited White Noise  Cov=[Position_noise]  Ts=0.1  seed=[23341]
  Demux : Demux  Outputs=7
  Mux : Mux  Inputs=7
  sensor_positions : Outport
  wires:
  Band-Limited White Noise2/1 -> Add2/1
  Band-Limited White Noise6/1 -> Add6/1
  Band-Limited White Noise1/1 -> Add1/1
  Band-Limited White Noise5/1 -> Add5/1
  Add5/1 -> Mux/6
  Demux/3 -> Add2/2
  Add3/1 -> Mux/4
  Add2/1 -> Mux/3
  Add1/1 -> Mux/2
  Mux/1 -> sensor_positions/1
  Add6/1 -> Mux/7
  Band-Limited White Noise/1 -> Add/1
  Demux/1 -> Add/2
  Demux/7 -> Add6/2
  Band-Limited White Noise3/1 -> Add3/1
  Demux/6 -> Add5/2
  Add/1 -> Mux/1
  Position/1 -> Demux/1
  Demux/2 -> Add1/2
  Demux/4 -> Add3/2
  Band-Limited White Noise4/1 -> Add4/1
  Demux/5 -> Add4/2
  Add4/1 -> Mux/5

== system simLink_linefollower/Control/Add and scale sensor values ==
  Sensor values : Inport
  Sensor_close values : Inport  Port=2
  Add and scale sensor : Subsystem
  Add and scale sensor_close : Subsystem
  Sensor sum : Outport
  Sensor_close sum : Outport  Port=2
  wires:
  Sensor_close values/1 -> Add and scale sensor_close/1(In1)
  Sensor values/1 -> Add and scale sensor/1(In1)
  Add and scale sensor/1(Out1) -> Sensor sum/1
  Add and scale sensor_close/1(Out1) -> Sensor_close sum/1

== system simLink_linefollower/All sensors pos/Sensor 1/Subsystem ==
  theta : Inport
  x : Inport  Port=2
  gain : Inport  Port=3
  sign : Inport  Port=4
  Add10 : Sum
  Constant10 : Constant  Value=pi/2
  Cos10 : Trigonometry  Operator=cos
  Product : Product  Inputs=4
  Subtract10 : Sum
  spacing : Constant  Value=spacing
  x_pos : Outport
  wires:
  Subtract10/1 -> Cos10/1
  Add10/1 -> x_pos/1
  Constant10/1 -> Subtract10/2
  x/1 -> Subtract10/1
  theta/1 -> Add10/1
  Product/1 -> Add10/2
  Cos10/1 -> Product/1
  gain/1 -> Product/2
  sign/1 -> Product/3
  spacing/1 -> Product/4

== system simLink_linefollower/All sensors pos/Sensor 1/Subsystem1 ==
  y : Inport
  theta : Inport  Port=2
  gain : Inport  Port=3
  sign : Inport  Port=4
  Add11 : Sum
  Constant11 : Constant  Value=pi/2
  Cos11 : Trigonometry
  Product : Product  Inputs=4
  Subtract11 : Sum
  spacing : Constant  Value=spacing
  y_pos : Outport
  wires:
  Subtract11/1 -> Cos11/1
  Constant11/1 -> Subtract11/2
  y/1 -> Add11/1
  Cos11/1 -> Product/1
  Add11/1 -> y_pos/1
  Product/1 -> Add11/2
  theta/1 -> Subtract11/1
  sign/1 -> Product/3
  gain/1 -> Product/2
  spacing/1 -> Product/4

== system simLink_linefollower/All sensors pos/Sensor 2/Subsystem ==
  theta : Inport
  x : Inport  Port=2
  gain : Inport  Port=3
  sign : Inport  Port=4
  Add10 : Sum
  Constant10 : Constant  Value=pi/2
  Cos10 : Trigonometry  Operator=cos
  Product : Product  Inputs=4
  Subtract10 : Sum
  spacing : Constant  Value=spacing
  x_pos : Outport
  wires:
  Subtract10/1 -> Cos10/1
  Add10/1 -> x_pos/1
  Constant10/1 -> Subtract10/2
  x/1 -> Subtract10/1
  theta/1 -> Add10/1
  Product/1 -> Add10/2
  Cos10/1 -> Product/1
  gain/1 -> Product/2
  sign/1 -> Product/3
  spacing/1 -> Product/4

== system simLink_linefollower/All sensors pos/Sensor 2/Subsystem1 ==
  y : Inport
  theta : Inport  Port=2
  gain : Inport  Port=3
  sign : Inport  Port=4
  Add11 : Sum
  Constant11 : Constant  Value=pi/2
  Cos11 : Trigonometry
  Product : Product  Inputs=4
  Subtract11 : Sum
  spacing : Constant  Value=spacing
  y_pos : Outport
  wires:
  Subtract11/1 -> Cos11/1
  Constant11/1 -> Subtract11/2
  y/1 -> Add11/1
  Cos11/1 -> Product/1
  Add11/1 -> y_pos/1
  Product/1 -> Add11/2
  theta/1 -> Subtract11/1
  sign/1 -> Product/3
  gain/1 -> Product/2
  spacing/1 -> Product/4

== system simLink_linefollower/All sensors pos/Sensor 3/Subsystem ==
  theta : Inport
  x : Inport  Port=2
  gain : Inport  Port=3
  sign : Inport  Port=4
  Add10 : Sum
  Constant10 : Constant  Value=pi/2
  Cos10 : Trigonometry  Operator=cos
  Product : Product  Inputs=4
  Subtract10 : Sum
  spacing : Constant  Value=spacing
  x_pos : Outport
  wires:
  Subtract10/1 -> Cos10/1
  Add10/1 -> x_pos/1
  Constant10/1 -> Subtract10/2
  x/1 -> Subtract10/1
  theta/1 -> Add10/1
  Product/1 -> Add10/2
  Cos10/1 -> Product/1
  gain/1 -> Product/2
  sign/1 -> Product/3
  spacing/1 -> Product/4

== system simLink_linefollower/All sensors pos/Sensor 3/Subsystem1 ==
  y : Inport
  theta : Inport  Port=2
  gain : Inport  Port=3
  sign : Inport  Port=4
  Add11 : Sum
  Constant11 : Constant  Value=pi/2
  Cos11 : Trigonometry
  Product : Product  Inputs=4
  Subtract11 : Sum
  spacing : Constant  Value=spacing
  y_pos : Outport
  wires:
  Subtract11/1 -> Cos11/1
  Constant11/1 -> Subtract11/2
  y/1 -> Add11/1
  Cos11/1 -> Product/1
  Add11/1 -> y_pos/1
  Product/1 -> Add11/2
  theta/1 -> Subtract11/1
  sign/1 -> Product/3
  gain/1 -> Product/2
  spacing/1 -> Product/4

== system simLink_linefollower/All sensors pos/Sensor 5/Subsystem ==
  theta : Inport
  x : Inport  Port=2
  gain : Inport  Port=3
  sign : Inport  Port=4
  Add10 : Sum
  Constant10 : Constant  Value=pi/2
  Cos10 : Trigonometry  Operator=cos
  Product : Product  Inputs=4
  Subtract10 : Sum
  spacing : Constant  Value=spacing
  x_pos : Outport
  wires:
  Subtract10/1 -> Cos10/1
  Add10/1 -> x_pos/1
  Constant10/1 -> Subtract10/2
  x/1 -> Subtract10/1
  theta/1 -> Add10/1
  Product/1 -> Add10/2
  Cos10/1 -> Product/1
  gain/1 -> Product/2
  sign/1 -> Product/3
  spacing/1 -> Product/4

== system simLink_linefollower/All sensors pos/Sensor 5/Subsystem1 ==
  y : Inport
  theta : Inport  Port=2
  gain : Inport  Port=3
  sign : Inport  Port=4
  Add11 : Sum
  Constant11 : Constant  Value=pi/2
  Cos11 : Trigonometry
  Product : Product  Inputs=4
  Subtract11 : Sum
  spacing : Constant  Value=spacing
  y_pos : Outport
  wires:
  Subtract11/1 -> Cos11/1
  Constant11/1 -> Subtract11/2
  y/1 -> Add11/1
  Cos11/1 -> Product/1
  Add11/1 -> y_pos/1
  Product/1 -> Add11/2
  theta/1 -> Subtract11/1
  sign/1 -> Product/3
  gain/1 -> Product/2
  spacing/1 -> Product/4

== system simLink_linefollower/All sensors pos/Sensor 6/Subsystem ==
  theta : Inport
  x : Inport  Port=2
  gain : Inport  Port=3
  sign : Inport  Port=4
  Add10 : Sum
  Constant10 : Constant  Value=pi/2
  Cos10 : Trigonometry  Operator=cos
  Product : Product  Inputs=4
  Subtract10 : Sum
  spacing : Constant  Value=spacing
  x_pos : Outport
  wires:
  Subtract10/1 -> Cos10/1
  Add10/1 -> x_pos/1
  Constant10/1 -> Subtract10/2
  x/1 -> Subtract10/1
  theta/1 -> Add10/1
  Product/1 -> Add10/2
  Cos10/1 -> Product/1
  gain/1 -> Product/2
  sign/1 -> Product/3
  spacing/1 -> Product/4

== system simLink_linefollower/All sensors pos/Sensor 6/Subsystem1 ==
  y : Inport
  theta : Inport  Port=2
  gain : Inport  Port=3
  sign : Inport  Port=4
  Add11 : Sum
  Constant11 : Constant  Value=pi/2
  Cos11 : Trigonometry
  Product : Product  Inputs=4
  Subtract11 : Sum
  spacing : Constant  Value=spacing
  y_pos : Outport
  wires:
  Subtract11/1 -> Cos11/1
  Constant11/1 -> Subtract11/2
  y/1 -> Add11/1
  Cos11/1 -> Product/1
  Add11/1 -> y_pos/1
  Product/1 -> Add11/2
  theta/1 -> Subtract11/1
  sign/1 -> Product/3
  gain/1 -> Product/2
  spacing/1 -> Product/4

== system simLink_linefollower/All sensors pos/Sensor 7/Subsystem ==
  theta : Inport
  x : Inport  Port=2
  gain : Inport  Port=3
  sign : Inport  Port=4
  Add10 : Sum
  Constant10 : Constant  Value=pi/2
  Cos10 : Trigonometry  Operator=cos
  Product : Product  Inputs=4
  Subtract10 : Sum
  spacing : Constant  Value=spacing
  x_pos : Outport
  wires:
  Subtract10/1 -> Cos10/1
  Add10/1 -> x_pos/1
  Constant10/1 -> Subtract10/2
  x/1 -> Subtract10/1
  theta/1 -> Add10/1
  Product/1 -> Add10/2
  Cos10/1 -> Product/1
  gain/1 -> Product/2
  sign/1 -> Product/3
  spacing/1 -> Product/4

== system simLink_linefollower/All sensors pos/Sensor 7/Subsystem1 ==
  y : Inport
  theta : Inport  Port=2
  gain : Inport  Port=3
  sign : Inport  Port=4
  Add11 : Sum
  Constant11 : Constant  Value=pi/2
  Cos11 : Trigonometry
  Product : Product  Inputs=4
  Subtract11 : Sum
  spacing : Constant  Value=spacing
  y_pos : Outport
  wires:
  Subtract11/1 -> Cos11/1
  Constant11/1 -> Subtract11/2
  y/1 -> Add11/1
  Cos11/1 -> Product/1
  Add11/1 -> y_pos/1
  Product/1 -> Add11/2
  theta/1 -> Subtract11/1
  sign/1 -> Product/3
  gain/1 -> Product/2
  spacing/1 -> Product/4

== system simLink_linefollower/All sensors_close pos/Sensor 1/Subsystem ==
  theta : Inport
  x : Inport  Port=2
  gain : Inport  Port=3
  sign : Inport  Port=4
  Add10 : Sum
  Constant10 : Constant  Value=pi/2
  Cos10 : Trigonometry  Operator=cos
  Product : Product  Inputs=4
  Subtract10 : Sum
  spacing : Constant  Value=spacing
  x_pos : Outport
  wires:
  Subtract10/1 -> Cos10/1
  Add10/1 -> x_pos/1
  Constant10/1 -> Subtract10/2
  x/1 -> Subtract10/1
  theta/1 -> Add10/1
  Product/1 -> Add10/2
  Cos10/1 -> Product/1
  gain/1 -> Product/2
  sign/1 -> Product/3
  spacing/1 -> Product/4

== system simLink_linefollower/All sensors_close pos/Sensor 1/Subsystem1 ==
  y : Inport
  theta : Inport  Port=2
  gain : Inport  Port=3
  sign : Inport  Port=4
  Add11 : Sum
  Constant11 : Constant  Value=pi/2
  Cos11 : Trigonometry
  Product : Product  Inputs=4
  Subtract11 : Sum
  spacing : Constant  Value=spacing
  y_pos : Outport
  wires:
  Subtract11/1 -> Cos11/1
  Constant11/1 -> Subtract11/2
  y/1 -> Add11/1
  Cos11/1 -> Product/1
  Add11/1 -> y_pos/1
  Product/1 -> Add11/2
  theta/1 -> Subtract11/1
  sign/1 -> Product/3
  gain/1 -> Product/2
  spacing/1 -> Product/4

== system simLink_linefollower/All sensors_close pos/Sensor 2/Subsystem ==
  theta : Inport
  x : Inport  Port=2
  gain : Inport  Port=3
  sign : Inport  Port=4
  Add10 : Sum
  Constant10 : Constant  Value=pi/2
  Cos10 : Trigonometry  Operator=cos
  Product : Product  Inputs=4
  Subtract10 : Sum
  spacing : Constant  Value=spacing
  x_pos : Outport
  wires:
  Subtract10/1 -> Cos10/1
  Add10/1 -> x_pos/1
  Constant10/1 -> Subtract10/2
  x/1 -> Subtract10/1
  theta/1 -> Add10/1
  Product/1 -> Add10/2
  Cos10/1 -> Product/1
  gain/1 -> Product/2
  sign/1 -> Product/3
  spacing/1 -> Product/4

== system simLink_linefollower/All sensors_close pos/Sensor 2/Subsystem1 ==
  y : Inport
  theta : Inport  Port=2
  gain : Inport  Port=3
  sign : Inport  Port=4
  Add11 : Sum
  Constant11 : Constant  Value=pi/2
  Cos11 : Trigonometry
  Product : Product  Inputs=4
  Subtract11 : Sum
  spacing : Constant  Value=spacing
  y_pos : Outport
  wires:
  Subtract11/1 -> Cos11/1
  Constant11/1 -> Subtract11/2
  y/1 -> Add11/1
  Cos11/1 -> Product/1
  Add11/1 -> y_pos/1
  Product/1 -> Add11/2
  theta/1 -> Subtract11/1
  sign/1 -> Product/3
  gain/1 -> Product/2
  spacing/1 -> Product/4

== system simLink_linefollower/All sensors_close pos/Sensor 3/Subsystem ==
  theta : Inport
  x : Inport  Port=2
  gain : Inport  Port=3
  sign : Inport  Port=4
  Add10 : Sum
  Constant10 : Constant  Value=pi/2
  Cos10 : Trigonometry  Operator=cos
  Product : Product  Inputs=4
  Subtract10 : Sum
  spacing : Constant  Value=spacing
  x_pos : Outport
  wires:
  Subtract10/1 -> Cos10/1
  Add10/1 -> x_pos/1
  Constant10/1 -> Subtract10/2
  x/1 -> Subtract10/1
  theta/1 -> Add10/1
  Product/1 -> Add10/2
  Cos10/1 -> Product/1
  gain/1 -> Product/2
  sign/1 -> Product/3
  spacing/1 -> Product/4

== system simLink_linefollower/All sensors_close pos/Sensor 3/Subsystem1 ==
  y : Inport
  theta : Inport  Port=2
  gain : Inport  Port=3
  sign : Inport  Port=4
  Add11 : Sum
  Constant11 : Constant  Value=pi/2
  Cos11 : Trigonometry
  Product : Product  Inputs=4
  Subtract11 : Sum
  spacing : Constant  Value=spacing
  y_pos : Outport
  wires:
  Subtract11/1 -> Cos11/1
  Constant11/1 -> Subtract11/2
  y/1 -> Add11/1
  Cos11/1 -> Product/1
  Add11/1 -> y_pos/1
  Product/1 -> Add11/2
  theta/1 -> Subtract11/1
  sign/1 -> Product/3
  gain/1 -> Product/2
  spacing/1 -> Product/4

== system simLink_linefollower/All sensors_close pos/Sensor 5/Subsystem ==
  theta : Inport
  x : Inport  Port=2
  gain : Inport  Port=3
  sign : Inport  Port=4
  Add10 : Sum
  Constant10 : Constant  Value=pi/2
  Cos10 : Trigonometry  Operator=cos
  Product : Product  Inputs=4
  Subtract10 : Sum
  spacing : Constant  Value=spacing
  x_pos : Outport
  wires:
  Subtract10/1 -> Cos10/1
  Add10/1 -> x_pos/1
  Constant10/1 -> Subtract10/2
  x/1 -> Subtract10/1
  theta/1 -> Add10/1
  Product/1 -> Add10/2
  Cos10/1 -> Product/1
  gain/1 -> Product/2
  sign/1 -> Product/3
  spacing/1 -> Product/4

== system simLink_linefollower/All sensors_close pos/Sensor 5/Subsystem1 ==
  y : Inport
  theta : Inport  Port=2
  gain : Inport  Port=3
  sign : Inport  Port=4
  Add11 : Sum
  Constant11 : Constant  Value=pi/2
  Cos11 : Trigonometry
  Product : Product  Inputs=4
  Subtract11 : Sum
  spacing : Constant  Value=spacing
  y_pos : Outport
  wires:
  Subtract11/1 -> Cos11/1
  Constant11/1 -> Subtract11/2
  y/1 -> Add11/1
  Cos11/1 -> Product/1
  Add11/1 -> y_pos/1
  Product/1 -> Add11/2
  theta/1 -> Subtract11/1
  sign/1 -> Product/3
  gain/1 -> Product/2
  spacing/1 -> Product/4

== system simLink_linefollower/All sensors_close pos/Sensor 6/Subsystem ==
  theta : Inport
  x : Inport  Port=2
  gain : Inport  Port=3
  sign : Inport  Port=4
  Add10 : Sum
  Constant10 : Constant  Value=pi/2
  Cos10 : Trigonometry  Operator=cos
  Product : Product  Inputs=4
  Subtract10 : Sum
  spacing : Constant  Value=spacing
  x_pos : Outport
  wires:
  Subtract10/1 -> Cos10/1
  Add10/1 -> x_pos/1
  Constant10/1 -> Subtract10/2
  x/1 -> Subtract10/1
  theta/1 -> Add10/1
  Product/1 -> Add10/2
  Cos10/1 -> Product/1
  gain/1 -> Product/2
  sign/1 -> Product/3
  spacing/1 -> Product/4

== system simLink_linefollower/All sensors_close pos/Sensor 6/Subsystem1 ==
  y : Inport
  theta : Inport  Port=2
  gain : Inport  Port=3
  sign : Inport  Port=4
  Add11 : Sum
  Constant11 : Constant  Value=pi/2
  Cos11 : Trigonometry
  Product : Product  Inputs=4
  Subtract11 : Sum
  spacing : Constant  Value=spacing
  y_pos : Outport
  wires:
  Subtract11/1 -> Cos11/1
  Constant11/1 -> Subtract11/2
  y/1 -> Add11/1
  Cos11/1 -> Product/1
  Add11/1 -> y_pos/1
  Product/1 -> Add11/2
  theta/1 -> Subtract11/1
  sign/1 -> Product/3
  gain/1 -> Product/2
  spacing/1 -> Product/4

== system simLink_linefollower/All sensors_close pos/Sensor 7/Subsystem ==
  theta : Inport
  x : Inport  Port=2
  gain : Inport  Port=3
  sign : Inport  Port=4
  Add10 : Sum
  Constant10 : Constant  Value=pi/2
  Cos10 : Trigonometry  Operator=cos
  Product : Product  Inputs=4
  Subtract10 : Sum
  spacing : Constant  Value=spacing
  x_pos : Outport
  wires:
  Subtract10/1 -> Cos10/1
  Add10/1 -> x_pos/1
  Constant10/1 -> Subtract10/2
  x/1 -> Subtract10/1
  theta/1 -> Add10/1
  Product/1 -> Add10/2
  Cos10/1 -> Product/1
  gain/1 -> Product/2
  sign/1 -> Product/3
  spacing/1 -> Product/4

== system simLink_linefollower/All sensors_close pos/Sensor 7/Subsystem1 ==
  y : Inport
  theta : Inport  Port=2
  gain : Inport  Port=3
  sign : Inport  Port=4
  Add11 : Sum
  Constant11 : Constant  Value=pi/2
  Cos11 : Trigonometry
  Product : Product  Inputs=4
  Subtract11 : Sum
  spacing : Constant  Value=spacing
  y_pos : Outport
  wires:
  Subtract11/1 -> Cos11/1
  Constant11/1 -> Subtract11/2
  y/1 -> Add11/1
  Cos11/1 -> Product/1
  Add11/1 -> y_pos/1
  Product/1 -> Add11/2
  theta/1 -> Subtract11/1
  sign/1 -> Product/3
  gain/1 -> Product/2
  spacing/1 -> Product/4

== system simLink_linefollower/Control/Add and scale sensor values/Add and scale sensor ==
  In1 : Inport
  Add : Sum  Inputs=+++++++
  Demux : Demux  Outputs=7
  Gain : Gain  Gain=-1
  Gain1 : Gain  Gain=0
  Gain2 : Gain
  Gain3 : Gain  Gain=2
  Gain4 : Gain  Gain=-3
  Gain5 : Gain  Gain=-2
  Gain6 : Gain  Gain=3
  Out1 : Outport
  wires:
  Demux/3 -> Gain/1
  Demux/7 -> Gain6/1
  Gain3/1 -> Add/6
  Gain5/1 -> Add/2
  Add/1 -> Out1/1
  Demux/6 -> Gain3/1
  Demux/5 -> Gain2/1
  Gain2/1 -> Add/5
  Gain1/1 -> Add/4
  Demux/4 -> Gain1/1
  Gain6/1 -> Add/7
  Gain4/1 -> Add/1
  Gain/1 -> Add/3
  In1/1 -> Demux/1
  Demux/2 -> Gain5/1
  Demux/1 -> Gain4/1

== system simLink_linefollower/Control/Add and scale sensor values/Add and scale sensor_close ==
  In1 : Inport
  Add : Sum  Inputs=+++++++
  Demux : Demux  Outputs=7
  Gain : Gain  Gain=-1
  Gain1 : Gain  Gain=0
  Gain2 : Gain
  Gain3 : Gain  Gain=2
  Gain4 : Gain  Gain=-3
  Gain5 : Gain  Gain=-2
  Gain6 : Gain  Gain=3
  Out1 : Outport
  wires:
  Demux/3 -> Gain/1
  Demux/7 -> Gain6/1
  Gain3/1 -> Add/6
  Gain5/1 -> Add/2
  Add/1 -> Out1/1
  Demux/6 -> Gain3/1
  Demux/5 -> Gain2/1
  Gain2/1 -> Add/5
  Gain1/1 -> Add/4
  Demux/4 -> Gain1/1
  Gain6/1 -> Add/7
  Gain4/1 -> Add/1
  Gain/1 -> Add/3
  In1/1 -> Demux/1
  Demux/2 -> Gain5/1
  Demux/1 -> Gain4/1
